simulink model "BANSHEE"  (Simulink 8.1)
settings: Solver=ode1  StartTime=0.0  StopTime=inf  FixedStep=Ts  MaxStep=1e-3  RelTol=1e-3
model workspace (MAT data in the model file):
  op_snapshot1 : opcond.OperatingPoint (value not decoded)
PostLoadFcn:
  | BANSHEE_init;
InitFcn:
  | BANSHEE_init;
values from neighbouring files (symbols this model uses):
  Ts = 100E-6    (= 0.0001)    [BANSHEE_init.m]
undefined symbols (not defined in the file or in its folder): Banshee_HWCtrl_IOs, Banshee_SEL751_Woodward_lib, DMS_slave_lib, DMSCommands, F1, F2, F3, fdesignblkfcn, Feeder1_lib, Feeder2_lib, Feeder3_lib, gcbh, generic_ethernet_cb, Left, relay_housing_lib, SM_UtilityService, SS_F1_RELAY_HOUSING, SS_F2_RELAY_HOUSING, SS_F3_RELAY_HOUSING, SS_Feeder1, SS_Feeder2, SS_Feeder3, TestSeq_slave_lib, TestSequenceCommands, type, utility_service_lib, V
libraries: breaker_lib x51, cables_lib x49, rtio_generic_modbus x45, relay_modbus_lib x42, transformer_lib x25, rtlab x23, simulink x23, Load_lib x20, powerlib x19, ssn_lib x17, rtio_opalrt_common x13, rtio_opalrt_op5142ex1 x12
(part 1 of 6)
settings Model: ARTEMISmethode_block_infos=$$__separator__$$BANSHEE/ARTEMIS Guide$$__separator__$$  Creator=RE25624  LastModifiedBy=re25624  BufferReuse=off
settings SolverCC: ZeroCrossAlgorithm=Adaptive
settings DataIOCC: ExternalInput=getinputstruct(op_snapshot1)  InitialState=getstatestruct(op_snapshot1)  LimitDataPoints=off  MaxDataPoints=90060  SignalLoggingSaveFormat=Dataset  SaveOutput=off  SignalLogging=off  DSMLogging=off  SaveTime=off  OutputSaveName=result
settings OptimizationCC: BlockReduction=off  OptimizeBlockIOStorage=off  BufferReuse=off  ExpressionFolding=off  LocalBlockOutputs=off
settings DebuggingCC: MaxConsecutiveZCsMsg=warning  IgnoredZcDiagnostic=none  SolverPrmCheckMsg=none  MultiTaskRateTransMsg=warning  FcnCallInpInsideContextMsg=EnableAllAsWarning  FrameProcessingCompatibilityMsg=error  ModelReferenceExtraNoncontSigs=warning  StrictBusMsg=None
settings ModelReferenceCC: UpdateModelReferenceTargets=IfOutOfDate
settings SFSimCC: SFSimEcho=off
settings GRTTargetCC: CodeReplacementLibrary=C89/C90 (ANSI)

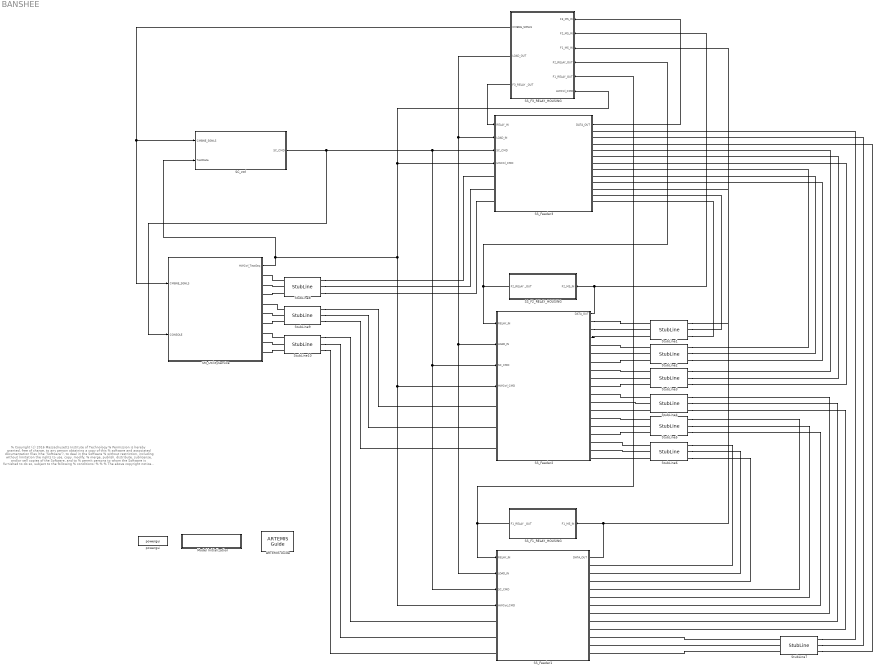
== system BANSHEE ==
  note: % Copyright (c) 2016 Massachusetts Institute of Technology
      | % Permission is hereby granted, free of charge, to any person obtaining a copy of this
      | % software and associated documentation files (the "Software"), to deal in the Software
      | % without restriction, including without limitation the rights to use, copy, modify,
      | % merge, publish, distribute, sublicense, and/or sell copies of the Software, and to
      | % permit persons to whom the Software is furnished to do so, subject to the following
      | % conditions:
      | %
      | %
      | % The above copyright notice and this permission notice shall be included in
      | % all copies or substantial portions of the Software.
      | %
      | % THE SOFTWARE IS PROVIDED "AS IS", WITHOUT WARRANTY OF ANY KIND, EXPRESS OR IMPLIED,
      | % INCLUDING BUT NOT LIMITED TO THE WARRANTIES OF MERCHANTABILITY, FITNESS FOR A
      | % PARTICULAR PURPOSE AND NONINFRINGEMENT. IN NO EVENT SHALL THE AUTHORS OR COPYRIGHT
      | % HOLDERS BE LIABLE FOR ANY CLAIM, DAMAGES OR OTHER LIABILITY, WHETHER IN AN ACTION
      | % OF CONTRACT, TORT OR OTHERWISE, ARISING FROM, OUT OF OR IN CONNECTION WITH THE
      | % SOFTWARE OR THE USE OR OTHER DEALINGS IN THE SOFTWARE.
      | %
      | %
      | %%
  ARTEMIS Guide : artemis/ARTEMIS/ARTEMIS Guide  Tag=FTSSmethode_opal_4hx0r99  Description=5.0_z1  lock=on  Ts=Ts  opt=art5  dyna=off  nb_perm=4  RT_fullcomp=off  ssn=on  ssn_itvc=off  ssn_ivic=off  ssn_ext=off  ssn_solver=Art5 with Backward Euler nodal interface  ssn_impulse=off  ssn_quasimpulse=off  ssn_impulse_loop=5  paraExtinctionThy=off  Thy_Impulse=on  dtc=Off  dtc_opt=normal  ao=on  simtype=off  ct_mac=off  lin_mov=off  lsp=[0.001 2]  spike_skip=Disabled  dtc_extra=1  dtc_sws=normal  dtc_pied=0.5  SPSRulesBlock=SPSRules  tre=on  ctmm=off  LF=off  dpl_type=ARTEMiS DPL  rlc_type=off  custom_type=off  para=on  ssn_ImpulseLoopBlockedStateUpdate=5  ssn_mov_iter_number=5  ssn_switch_iter_number=5
  Model Initialization : Subsystem  AncestorBlock=artemis/Tools /Misc/Model Initialization  mask(Model Functions){InitFcnX=BANSHEE_init;, prel=off, posl=on, inif=on, strf=off}
      mask prompts: InitFcnX "Initialisation"; prel "Preload Function"; posl "PostLoad Function"; inif "InitFcn"; strf "StartFcn"
      mask init:
      | currentBlock = gcb;
      | root = bdroot(currentBlock);
      | 
      | if ~strcmp(get_param(root,'BlockDiagramType'),'library')
      |     if prel==1
      |         set_param(root, 'PreLoadFcn', InitFcnX);
      |     else
      |         set_param(root, 'PreLoadFcn', '');
      |     end
      |     if inif==1
      |         set_param(root, 'InitFcn', InitFcnX);
      |     else
      |         set_param(root, 'InitFcn', '');
      |     end
      |     if strf==1
      |         set_param(root, 'StartFcn', InitFcnX);
      |     else
      |         set_param(root, 'StartFcn', '');
      |     end
      |     if posl==1
      |         set_param(root, 'PostLoadFcn', InitFcnX);
      |     else
      |         set_param(root, 'PostLoadFcn', '');
      |     end
      | end
      | 
      | pos = get_param(currentBlock, 'Position');
      | width = pos(3) - pos(1); height = pos(4) - pos(2);
      | txt = [ upper(root) '\n' '- InitFcn. . . . . '  get_param(root, 'InitFcn') ];
      settings: CopyFcn=set_param(gcb,'LinkStatus','inactive')
      mask Display: text(5, height*0.5, txt, 'horizontalAlignment', 'left', 'verticalAlignment', 'middle') ;
  SC_ctrl : Subsystem
  SM_UtilityService : Subsystem  AncestorBlock=utility_service_lib/SM_UtilityService
  SS_F1_RELAY_HOUSING : Subsystem  AncestorBlock=relay_housing_lib/SS_F1_RELAY_HOUSING
  SS_F2_RELAY_HOUSING : Subsystem  AncestorBlock=relay_housing_lib/SS_F2_RELAY_HOUSING
  SS_F3_RELAY_HOUSING : Subsystem  AncestorBlock=relay_housing_lib/SS_F3_RELAY_HOUSING
  SS_Feeder1 : Subsystem  AncestorBlock=Feeder1_lib/SS_Feeder1
  SS_Feeder2 : Subsystem  AncestorBlock=Feeder2_lib/SS_Feeder2
  SS_Feeder3 : Subsystem  AncestorBlock=Feeder3_lib/SS_Feeder3
  StubLine1 : artemis/ARTEMIS/StubLine  Phases=3  pu=off  L=1500 * 9.43453e-08 / 2  Lpu=0.08  R=1500 * 2.28409e-5 / 2  Rpu=0.002  S_base=450e6/3  V_base=230e3/sqrt(3)  F_base=60  Ts=Ts
  StubLine10 : artemis/ARTEMIS/StubLine  Phases=3  pu=on  L=1500 * 9.43453e-08 / 2  Lpu=0.08  R=1500 * 2.28409e-5 / 2  Rpu=0.002  S_base=50e6/3  V_base=13.8e3/sqrt(3)  F_base=60  Ts=Ts
  StubLine2 : artemis/ARTEMIS/StubLine  Phases=3  pu=off  L=1500 * 9.43453e-08 / 2  Lpu=0.08  R=1500 * 2.28409e-5 / 2  Rpu=0.002  S_base=450e6/3  V_base=230e3/sqrt(3)  F_base=60  Ts=Ts
  StubLine3 : artemis/ARTEMIS/StubLine  Phases=3  pu=off  L=1500 * 9.43453e-08 / 2  Lpu=0.08  R=1500 * 2.28409e-5 / 2  Rpu=0.002  S_base=450e6/3  V_base=230e3/sqrt(3)  F_base=60  Ts=Ts
  StubLine4 : artemis/ARTEMIS/StubLine  Phases=3  pu=off  L=1000 * 9.43453e-08 / 2  Lpu=0.08  R=1000 * 2.28409e-5 / 2  Rpu=0.002  S_base=450e6/3  V_base=230e3/sqrt(3)  F_base=60  Ts=Ts
  StubLine5 : artemis/ARTEMIS/StubLine  Phases=3  pu=off  L=2000 * 9.43453e-08 / 2  Lpu=0.08  R=2000 * 2.28409e-5 / 2  Rpu=0.002  S_base=450e6/3  V_base=230e3/sqrt(3)  F_base=60  Ts=Ts
  StubLine6 : artemis/ARTEMIS/StubLine  Phases=3  pu=off  L=3000 * 9.43453e-08 / 1  Lpu=0.08  R=3000 * 2.28409e-5 / 1  Rpu=0.002  S_base=450e6/3  V_base=230e3/sqrt(3)  F_base=60  Ts=Ts
  StubLine7 : artemis/ARTEMIS/StubLine  Phases=3  pu=off  L=2000 * 9.43453e-08 / 2  Lpu=0.08  R=2000 * 2.28409e-5 / 2  Rpu=0.002  S_base=450e6/3  V_base=230e3/sqrt(3)  F_base=60  Ts=Ts
  StubLine8 : artemis/ARTEMIS/StubLine  Phases=3  pu=on  L=1500 * 9.43453e-08 / 2  Lpu=0.08  R=1500 * 2.28409e-5 / 2  Rpu=0.002  S_base=50e6/3  V_base=13.8e3/sqrt(3)  F_base=60  Ts=Ts
  StubLine9 : artemis/ARTEMIS/StubLine  Phases=3  pu=on  L=1500 * 9.43453e-08 / 2  Lpu=0.08  R=1500 * 2.28409e-5 / 2  Rpu=0.002  S_base=50e6/3  V_base=13.8e3/sqrt(3)  F_base=60  Ts=Ts
  powergui : powerlib/powergui  Priority=2  SimulationMode=Discrete  SolverType=Tustin  SampleTime=Ts  frequency=60  SPID=off  DisableSnubberDevices=off  DisableRonSwitches=off  DisableVfSwitches=off  SwTol=0  Interpol=off  DisplayEquations=off  frequencyindice=0  Pbase=100e6  ErrMax=1e-4  Iterations=50  UnitsV=kV  UnitsW=MW  FunctionMessages=off  echomessages=off  HookPort=off  EnableUseOfTLC=off  x0status=blocks  RestoreLinks=warning  ResistiveCurrentMeasurement=off  Frange=logspace(0,3,50)  Ylog=off  Xlog=off  ShowGrid=off  save=off  variable=ZData  structure=0  ZoomFFT=on  StartTime=0.0  cycles=2  DisplayStyle=off  fundamental=60  FreqAxis=off  MaxFrequency=1000  frequencyindicesteady=1  RmsSteady=1  display=off  Ts=0  methode=off
  wires:
  SS_Feeder3/1(DATA_OUT) -> SS_F3_RELAY_HOUSING/1(F3_MS_IN)
  SS_F3_RELAY_HOUSING/3(F3_RELAY _OUT) -> SS_Feeder3/1(RELAY_IN)
  SS_F1_RELAY_HOUSING/1(F1_RELAY _OUT) -> SS_Feeder1/1(RELAY_IN), SS_F3_RELAY_HOUSING/5(F1_RELAY_OUT)
  SS_F2_RELAY_HOUSING/1(F2_RELAY _OUT) -> SS_F3_RELAY_HOUSING/4(F2_RELAY_OUT), SS_Feeder2/1(RELAY_IN)
  SS_Feeder1/1(DATA_OUT) -> SS_F3_RELAY_HOUSING/3(F1_MS_IN), SS_F1_RELAY_HOUSING/1(F1_MS_IN)
  SS_Feeder2/1(DATA_OUT) -> SS_F3_RELAY_HOUSING/2(F2_MS_IN), SS_F2_RELAY_HOUSING/1(F2_MS_IN)
  SS_F3_RELAY_HOUSING/2(LOAD_OUT) -> SS_Feeder1/2(LOAD_IN), SS_Feeder2/2(LOAD_IN), SS_Feeder3/2(LOAD_IN)
  SM_UtilityService/1(HWCtrl_TestSeq) -> SC_ctrl/2(TestData), SS_Feeder1/4(HWCtrl_CMD), SS_Feeder2/4(HWCtrl_CMD), SS_F3_RELAY_HOUSING/6(HWCtrl_CMD), SS_Feeder3/4(HWCtrl_CMD)
  SS_F3_RELAY_HOUSING/1(CMBNE_SGNLS) -> SM_UtilityService/1(CMBNE_SGNLS), SC_ctrl/1(CMBNE_SGNLS)
  SC_ctrl/1(SC_CMD) -> SS_Feeder1/3(SC_CMD), SS_Feeder2/3(SC_CMD), SS_Feeder3/3(SC_CMD), SM_UtilityService/2(CONSOLE)
  connections:
  SS_Feeder2/RConn2 -- StubLine1/LConn2
  SS_Feeder2/RConn1 -- StubLine1/LConn1
  SS_Feeder2/RConn3 -- StubLine1/LConn3
  StubLine2/LConn2 -- SS_Feeder2/RConn5
  StubLine2/LConn3 -- SS_Feeder2/RConn6
  StubLine2/LConn1 -- SS_Feeder2/RConn4
  StubLine3/LConn2 -- SS_Feeder2/RConn8
  StubLine3/LConn1 -- SS_Feeder2/RConn7
  StubLine3/LConn3 -- SS_Feeder2/RConn9
  StubLine4/LConn3 -- SS_Feeder2/RConn12
  StubLine4/LConn2 -- SS_Feeder2/RConn11
  StubLine4/LConn1 -- SS_Feeder2/RConn10
  StubLine7/LConn3 -- SS_Feeder1/RConn12
  StubLine7/LConn2 -- SS_Feeder1/RConn11
  StubLine7/LConn1 -- SS_Feeder1/RConn10
  StubLine5/LConn2 -- SS_Feeder2/RConn14
  StubLine5/LConn1 -- SS_Feeder2/RConn13
  StubLine5/LConn3 -- SS_Feeder2/RConn15
  StubLine6/LConn3 -- SS_Feeder2/RConn18
  StubLine6/LConn2 -- SS_Feeder2/RConn17
  StubLine6/LConn1 -- SS_Feeder2/RConn16
  StubLine6/RConn1 -- SS_Feeder1/RConn1
  StubLine6/RConn2 -- SS_Feeder1/RConn2
  StubLine6/RConn3 -- SS_Feeder1/RConn3
  StubLine5/RConn1 -- SS_Feeder1/RConn4
  StubLine5/RConn2 -- SS_Feeder1/RConn5
  StubLine5/RConn3 -- SS_Feeder1/RConn6
  StubLine4/RConn1 -- SS_Feeder1/RConn7
  StubLine4/RConn2 -- SS_Feeder1/RConn8
  StubLine4/RConn3 -- SS_Feeder1/RConn9
  StubLine3/RConn3 -- SS_Feeder3/RConn6
  StubLine3/RConn2 -- SS_Feeder3/RConn5
  StubLine3/RConn1 -- SS_Feeder3/RConn4
  StubLine2/RConn3 -- SS_Feeder3/RConn9
  StubLine2/RConn2 -- SS_Feeder3/RConn8
  StubLine2/RConn1 -- SS_Feeder3/RConn7
  StubLine1/RConn3 -- SS_Feeder3/RConn12
  StubLine1/RConn2 -- SS_Feeder3/RConn11
  StubLine1/RConn1 -- SS_Feeder3/RConn10
  StubLine7/RConn1 -- SS_Feeder3/RConn1
  StubLine7/RConn2 -- SS_Feeder3/RConn2
  StubLine7/RConn3 -- SS_Feeder3/RConn3
  StubLine8/LConn1 -- SM_UtilityService/RConn1
  StubLine8/LConn2 -- SM_UtilityService/RConn2
  StubLine8/LConn3 -- SM_UtilityService/RConn3
  StubLine9/LConn2 -- SM_UtilityService/RConn5
  StubLine9/LConn3 -- SM_UtilityService/RConn6
  StubLine9/LConn1 -- SM_UtilityService/RConn4
  StubLine10/LConn2 -- SM_UtilityService/RConn8
  StubLine10/LConn3 -- SM_UtilityService/RConn9
  StubLine10/LConn1 -- SM_UtilityService/RConn7
  StubLine8/RConn3 -- SS_Feeder3/LConn3
  StubLine8/RConn2 -- SS_Feeder3/LConn2
  StubLine8/RConn1 -- SS_Feeder3/LConn1
  StubLine10/RConn1 -- SS_Feeder1/LConn1
  StubLine10/RConn2 -- SS_Feeder1/LConn2
  StubLine10/RConn3 -- SS_Feeder1/LConn3
  StubLine9/RConn1 -- SS_Feeder2/LConn1
  StubLine9/RConn2 -- SS_Feeder2/LConn2
  StubLine9/RConn3 -- SS_Feeder2/LConn3

== system BANSHEE/Model Initialization ==

== system BANSHEE/SC_ctrl ==
  note: % Copyright (c) 2016 Massachusetts Institute of Technology
      | % Permission is hereby granted, free of charge, to any person obtaining a copy of this
      | % software and associated documentation files (the "Software"), to deal in the Software
      | % without restriction, including without limitation the rights to use, copy, modify,
      | % merge, publish, distribute, sublicense, and/or sell copies of the Software, and to
      | % permit persons to whom the Software is furnished to do so, subject to the following
      | % conditions:
      | %
      | %
      | % The above copyright notice and this permission notice shall be included in
      | % all copies or substantial portions of the Software.
      | %
      | % THE SOFTWARE IS PROVIDED "AS IS", WITHOUT WARRANTY OF ANY KIND, EXPRESS OR IMPLIED,
      | % INCLUDING BUT NOT LIMITED TO THE WARRANTIES OF MERCHANTABILITY, FITNESS FOR A
      | % PARTICULAR PURPOSE AND NONINFRINGEMENT. IN NO EVENT SHALL THE AUTHORS OR COPYRIGHT
      | % HOLDERS BE LIABLE FOR ANY CLAIM, DAMAGES OR OTHER LIABILITY, WHETHER IN AN ACTION
      | % OF CONTRACT, TORT OR OTHERWISE, ARISING FROM, OUT OF OR IN CONNECTION WITH THE
      | % SOFTWARE OR THE USE OR OTHER DEALINGS IN THE SOFTWARE.
      | %
      | %
      | %%
  CMBNE_SGNLS : Inport
  TestData : Inport  Port=2
  Bus Creator : BusCreator  Inputs=2
  Bus Creator1 : BusCreator  Inputs=5
  Bus Creator2 : BusCreator  Inputs=2
  Bus Creator3 : BusCreator  Inputs=5
  DO NOT WRITE : Constant  Value=0
  F1 1: connect motor 0: disconnect motor1 : Constant  Value=0
  F3 1: connect motor 0: disconnect motor : Constant  Value=0
  FAULT : Constant
  Grid_Status_Ctrl : Subsystem  mask(Grid Status Control){Substation=1, Grid_F1=1, Grid_F2=1, Grid_F3=1, useDTT=1}
      mask prompts: Substation "Substation On [1] - Off [0]"; Grid_F1 "Grid_F1 On [1] - Off [0]"; Grid_F2 "Grid_F2 On [1] - Off [0]"; Grid_F3 "Grid_F3 On [1] - Off [0]"; useDTT "DTT Active On [1] - Off [0]"
      mask help: Use this block to trip and reconnect the feeder breakers serving Banshee
  Manual Switch{,1..6} (7 alike) : ManualSwitch
  NO FAULT : Constant  Value=0
  OpComm : rtlab/OpComm  nbport=2  groupe_acq=1  subsys_rate=0  st=0  Synchronization=on  Interpolation=on  Threshold=1.0  Missed_Data=off  Sim_Time=off  Samples=off  dynSigOut=off  from_console=0  warning_done=off  writeOpCommFile=off  Offset=off
  Plots : Subsystem
  Status : Display
  TestSeq : Subsystem
  WRITE : Constant
  Woodward : Subsystem
  SC_CMD : Outport
  wires:
  CMBNE_SGNLS/1 -> OpComm/1
  Bus Creator1/1 -> SC_CMD/1
  [IO_ctrl] -> Bus Creator1/3  "IO ctrl"
  Woodward/1(IOctrl) -> [IO_ctrl]
  [fault_cmd] -> Bus Creator1/1  "fault_cmd"
  Bus Creator/1 -> Bus Creator1/2  "motor_ONOFF"
  F3 1: connect motor 0: disconnect motor/1 -> Bus Creator/1  "F3_motor_ONOFF"
  F1 1: connect motor 0: disconnect motor1/1 -> Bus Creator/2  "F1_motor_ONOFF"
  Grid_Status_Ctrl/1(o) -> Status/1, Bus Creator1/4  "GridStatusCtrl"
  Manual Switch/1 -> Bus Creator2/1  "record_rms_signals"
  Manual Switch1/1 -> Bus Creator2/2  "record_inst_signals"
  Bus Creator2/1 -> Bus Creator1/5  "DataLogging"
  OpComm/1 -> Plots/1(CMBNE_SGNLS)
  OpComm/2 -> TestSeq/1(TestData)
  TestData/1 -> OpComm/2
  WRITE/1 -> Manual Switch1/2, Manual Switch/2  "record_rms_signals"
  DO NOT WRITE/1 -> Manual Switch1/1, Manual Switch/1
  Bus Creator3/1 -> [fault_cmd]
  Manual Switch2/1 -> Bus Creator3/1  "fault_location_1"
  Manual Switch6/1 -> Bus Creator3/5  "fault_location_5"
  Manual Switch3/1 -> Bus Creator3/2  "fault_location_2"
  Manual Switch4/1 -> Bus Creator3/3  "fault_location_3"
  Manual Switch5/1 -> Bus Creator3/4  "fault_location_4"
  NO FAULT/1 -> Manual Switch6/1, Manual Switch5/1, Manual Switch4/1, Manual Switch3/1, Manual Switch2/1
  FAULT/1 -> Manual Switch2/2, Manual Switch6/2, Manual Switch5/2, Manual Switch4/2, Manual Switch3/2  "record_rms_signals"

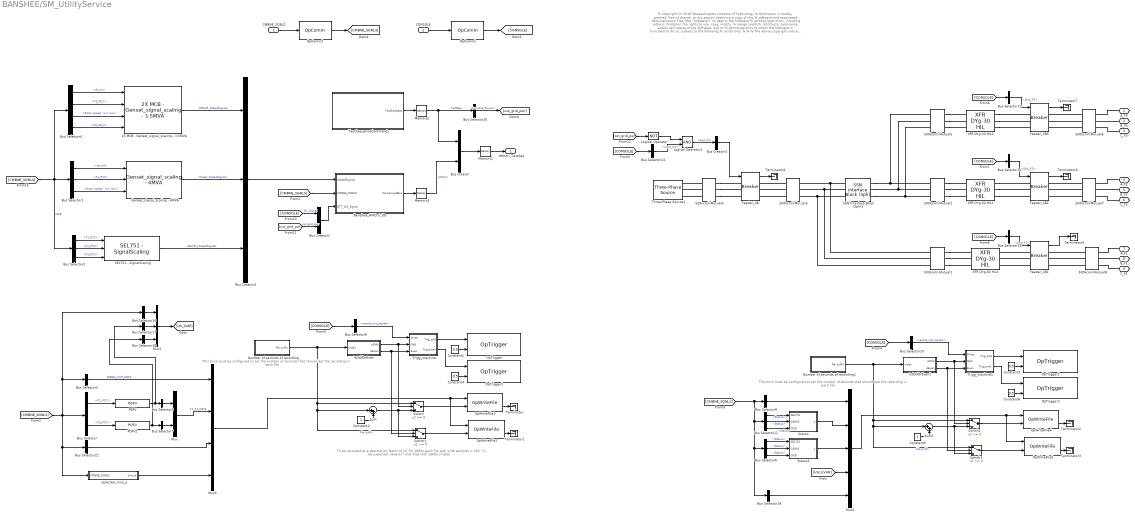
== system BANSHEE/SM_UtilityService ==
  note: % Copyright (c) 2016 Massachusetts Institute of Technology
      | % Permission is hereby granted, free of charge, to any person obtaining a copy of this
      | % software and associated documentation files (the "Software"), to deal in the Software
      | % without restriction, including without limitation the rights to use, copy, modify,
      | % merge, publish, distribute, sublicense, and/or sell copies of the Software, and to
      | % permit persons to whom the Software is furnished to do so, subject to the following
      | % conditions:
      | %
      | %
      | % The above copyright notice and this permission notice shall be included in
      | % all copies or substantial portions of the Software.
      | %
      | % THE SOFTWARE IS PROVIDED "AS IS", WITHOUT WARRANTY OF ANY KIND, EXPRESS OR IMPLIED,
      | % INCLUDING BUT NOT LIMITED TO THE WARRANTIES OF MERCHANTABILITY, FITNESS FOR A
      | % PARTICULAR PURPOSE AND NONINFRINGEMENT. IN NO EVENT SHALL THE AUTHORS OR COPYRIGHT
      | % HOLDERS BE LIABLE FOR ANY CLAIM, DAMAGES OR OTHER LIABILITY, WHETHER IN AN ACTION
      | % OF CONTRACT, TORT OR OTHERWISE, ARISING FROM, OUT OF OR IN CONNECTION WITH THE
      | % SOFTWARE OR THE USE OR OTHER DEALINGS IN THE SOFTWARE.
      | %
      | %
      | %%
  note: This bock must be configured to set the number of
      | seconds that should last the recording in each file
  note: To be recorded at a decimation factor of 10,   for 1800s each file with a Nb samples = 200.
      | To be expected: several *.mat files with 1800s of data
  note: This bock must be configured to set the number of
      | seconds that should last the recording in each file
  CMBNE_SGNLS : Inport
  CONSOLE : Inport  Port=2
  2X MCB - Genset_signal_scaling - 3.5MVA : EasyGen3500_GensetSignalScaling_lib/2X MCB - Genset_signal_scaling - 3.5MVA  Vpk_mcb=11268  watt_mcb=3150000  Vpk_gcb=11268  watt_gcb=3150000  rated_rpm=1800  wm_noise_bias=0.02
  500kcmil-Mutual1 : cables_lib/500kcmil-Mutual  length=200  par_sets=1  ratio=3
  500kcmil-Mutual2 : cables_lib/500kcmil-Mutual  length=200  par_sets=1  ratio=3
  500kcmil-Mutual{3..4,6..8} (5 alike) : cables_lib/500kcmil-Mutual  length=50  par_sets=1  ratio=3
  500kcmil-Mutual5 : cables_lib/500kcmil-Mutual  length=200  par_sets=1  ratio=3
  Banshee_HWCtrl_IOs : Subsystem  AncestorBlock=Banshee_SEL751_Woodward_lib/Banshee_HWCtrl_IOs
  Bus Creator : BusCreator  Inputs=2
  Bus Creator1 : BusCreator  Inputs=2
  Bus Creator2 : BusCreator  Inputs=1
  Bus Creator4 : BusCreator  Inputs=3
  Bus Selector : BusSelector  OutputSignals=F1_MS_IN.CB_DATA.F1_PCC,F3_MS_IN.CB_DATA.F3_PCC
  Bus Selector1 : BusSelector  OutputSignals="F1_MS_IN.DIESEL_DATA.DIESEL_GCB.cb_ms,F1_MS_IN.CB_DATA.F1_PCC,F1_MS_IN.DIESEL_DATA.Gen2_meas.w.w.Rotor speed  wm (pu)"
  Bus Selector10 : BusSelector  OutputSignals=DataLogging.record_inst_signals
  Bus Selector11 : BusSelector  OutputSignals=F1_MS_IN.CB_DATA.F1_PCC.Status,F1_MS_IN.CB_DATA.F1_CB_3.Status,F1_MS_IN.DIESEL_DATA.DIESEL_GCB.cb_ms.Status
  Bus Selector12 : BusSelector  OutputSignals=GridStatusCtrl.Substation.Logic_trip
  Bus Selector13 : BusSelector  OutputSignals=GridStatusCtrl.Grid_F3
  Bus Selector14 : BusSelector  OutputSignals=GridStatusCtrl.Grid_F2
  Bus Selector15 : BusSelector  OutputSignals=GridStatusCtrl.Grid_F1
  Bus Selector16 : BusSelector  OutputSignals=F1_MS_IN.DIESEL_DATA.DIESEL_GCB.kw,F1_MS_IN.DIESEL_DATA.DIESEL_GCB.kvar,F3_MS_IN.NG_CHP_DATA.NG_CHP_GCB.kw,F3_MS_IN.NG_CHP_DATA.NG_CHP_GCB.kvar  OutputAsBus=on
  Bus Selector17 : BusSelector  OutputSignals=kw,kvar  OutputAsBus=on
  Bus Selector18 : BusSelector  OutputSignals=kw,kvar  OutputAsBus=on
  Bus Selector19 : BusSelector  OutputSignals=F1_MS_IN.DIESEL_DATA.DIESEL_GCB.cb_ms.Iabc,F3_MS_IN.NG_CHP_DATA.NG_CHP_GCB.cb_ms.Iabc,F1_MS_IN.DIESEL_DATA.Gen2_meas.Vf.vf,F3_MS_IN.NG_CHP_DATA.Gen1_meas.Vf.vf  OutputAsBus=on
  Bus Selector2 : BusSelector  OutputSignals=F1_MS_IN.CB_DATA.F1_PCC,F2_MS_IN.CB_DATA.F2_PCC,F3_MS_IN.CB_DATA.F3_PCC
  Bus Selector20 : BusSelector  OutputSignals=Cut_Grid_Power
  Bus Selector21 : BusSelector  OutputSignals=F1_RELAY_OUT.F1_CB_1.m.status,F1_RELAY_OUT.F1_CB_2.m.status,F1_RELAY_OUT.F1_CB_3.m.status,F1_RELAY_OUT.F1_CB_4.m.status,F1_RELAY_OUT.F1_CB_5.m.status,F1_RELAY_OUT.F1_CB_6.m.status,F1_RELAY_OUT.F1_CB_7.m.status,F1_RELAY_OUT.F1_CB_8.m.status,F1_RELAY_OUT.F1_CB_9.m.status,F1_RELAY_OUT.F1_CB_10.m.status,F1_RELAY_OUT.F1_CB_11.m.status,F1_RELAY_OUT.F1_CB_12.m.status,F1_RELAY_OUT.F1_CB_13.m.status,F1_RELAY_OUT.F1_CB_14.m.status,F2_RELAY_OUT.F2_CB_1.m.status,F2_RELAY_OUT.F2_CB_2.m.status,F2_RELAY_OUT.F2_CB_3.m.status,F2_RELAY_OUT.F2_CB_4.m.status,F2_RELAY_OUT.F2_CB_5.m.status,F2_RELAY_OUT.F2_CB_6.m.status,F2_RELAY_OUT.F2_CB_7.m.status,F2_RELAY_OUT.F2_CB_8.m.status,F2_RELAY_OUT.F2_CB_9.m.status,F2_RELAY_OUT.F2_CB_10.m.status,F2_RELAY_OUT.F2_CB_11.m.status,F2_RELAY_OUT.F2_CB_12.m.status,F2_RELAY_OUT.F2_CB_13.m.status,F2_RELAY_OUT.F2_CB_14.m.status,F2_RELAY_OUT.F2_CB_15.m.status,F2_RELAY_OUT.F2_CB_16.m.status,F2_RELAY_OUT.F2_CB_17.m.status,F2_RELAY_OUT.F2_CB_18.m.status,F2_RELAY_OUT.F2_CB_19.m.status,F3_RELAY_OUT.F3_CB_1.m.status,F3_RELAY_OUT.F3_CB_2.m.status,F3_RELAY_OUT.F3_CB_3.m.status,F3_RELAY_OUT.F3_CB_4.m.status,F3_RELAY_OUT.F3_CB_5.m.status,F3_RELAY_OUT.F3_CB_6.m.status,F3_RELAY_OUT.F3_CB_7.m.status,F3_RELAY_OUT.F3_CB_8.m.status,F3_RELAY_OUT.F3_CB_9.m.status  OutputAsBus=on
  Bus Selector3 : BusSelector  OutputSignals=F1_MS_IN.DIESEL_DATA.DIESEL_GCB.VRMSLL,F1_MS_IN.DIESEL_DATA.DIESEL_GCB.Freq,F1_MS_IN.DIESEL_DATA.DIESEL_GCB.kw,F1_MS_IN.DIESEL_DATA.DIESEL_GCB.kvar,F3_MS_IN.NG_CHP_DATA.NG_CHP_GCB.VRMSLL,F3_MS_IN.NG_CHP_DATA.NG_CHP_GCB.Freq,F3_MS_IN.NG_CHP_DATA.NG_CHP_GCB.kw,F3_MS_IN.NG_CHP_DATA.NG_CHP_GCB.kvar  OutputAsBus=on
  Bus Selector4 : BusSelector  OutputSignals="F3_MS_IN.NG_CHP_DATA.NG_CHP_GCB.cb_ms,F3_MS_IN.CB_DATA.F3_PCC,F3_MS_IN.NG_CHP_DATA.Gen1_meas.w.w.Rotor speed  wm (pu),F3_MS_IN.CB_DATA.F3_CB_3"
  Bus Selector5 : BusSelector  OutputSignals=VRMSLL,Freq,kw,kvar  OutputAsBus=on
  Bus Selector6 : BusSelector  OutputSignals=F3_MS_IN.CB_DATA.F3_PCC.Status,F3_MS_IN.CB_DATA.F3_CB_3.Status,F3_MS_IN.NG_CHP_DATA.NG_CHP_GCB.cb_ms.Status
  Bus Selector7 : BusSelector  OutputSignals=VRMSLL,Freq,kw,kvar  OutputAsBus=on
  Bus Selector8 : BusSelector  OutputSignals=DataLogging.record_rms_signals
  Bus Selector9 : BusSelector  OutputSignals=F1_MS_IN.CB_DATA.F1_PCC.Vabc_bus,F3_MS_IN.CB_DATA.F3_PCC.Vabc_bus,F1_MS_IN.DIESEL_DATA.DIESEL_GCB.cb_ms.Vabc_bus,F3_MS_IN.NG_CHP_DATA.NG_CHP_GCB.cb_ms.Vabc_bus  OutputAsBus=on
  Constant{1,3..4,6} (4 alike) : Constant  Value=0.5
  Constant2 : Constant
  Constant5 : Constant
  Feeder_CB{,1..3} (4 alike) : breaker_lib/Breaker  Ts=Ts  mech_delay=cb_mech_delay
  Genset_signal_scaling - 4MVA : EasyGen3500_GensetSignalScaling_lib/Genset_signal_scaling - 4MVA  Vpk_mcb=11268  watt_mcb=3600000  Vpk_gcb=11268  watt_gcb=3600000  rated_rpm=1800  wm_noise_bias=0.02
  Logical Operator : Logic  Operator=NOT  AllPortsSameDT=off  OutDataTypeStr=boolean
  Logical Operator1 : Logic  AllPortsSameDT=off  OutDataTypeStr=boolean
  Memory1 : Memory
  Memory2 : Memory
  Memory3 : Memory
  Mux : Mux  Inputs=2
  Mux1 : Mux  Inputs=3
  Mux2 : Mux  Inputs=5
  Mux3 : Mux
  Number of seconds of recording : Subsystem  mask{time_s=1800}
      mask prompts: time_s "Time in seconds"
      mask help: Set the number of seconds that should last the recording in each file.
  Number of seconds of recording1 : Subsystem  mask{time_s=300}
      mask prompts: time_s "Time in seconds"
      mask help: Set the number of seconds that should last the recording in each file.
  OpComm1 : rtlab/OpComm  nbport=1  groupe_acq=1  subsys_rate=0  st=0  Synchronization=on  Interpolation=on  Threshold=1.0  Missed_Data=off  Sim_Time=off  Samples=off  dynSigOut=off  from_console=1  warning_done=off  writeOpCommFile=off  Offset=off
  OpComm2 : rtlab/OpComm  nbport=1  groupe_acq=1  subsys_rate=0  st=0  Synchronization=on  Interpolation=on  Threshold=1.0  Missed_Data=off  Sim_Time=off  Samples=off  dynSigOut=off  from_console=0  warning_done=off  writeOpCommFile=off  Offset=off
  OpTrigger : rtlab/DataLogging/OpTrigger  Trig_Type=TRIGGER SIGNAL >= TRIGGER LEVEL  Trig_Offset=0  Acq_Group=28
  OpTrigger1 : rtlab/DataLogging/OpTrigger  Trig_Type=TRIGGER SIGNAL >= TRIGGER LEVEL  Trig_Offset=0  Acq_Group=29
  OpTrigger2 : rtlab/DataLogging/OpTrigger  Trig_Type=TRIGGER SIGNAL >= TRIGGER LEVEL  Trig_Offset=0  Acq_Group=26
  OpTrigger3 : rtlab/DataLogging/OpTrigger  Trig_Type=TRIGGER SIGNAL >= TRIGGER LEVEL  Trig_Offset=0  Acq_Group=27
  OpWriteFile1 : rtlab/DataLogging/OpWriteFile  Static_File=off  varname=recVar  Filename=A_FILE_RECORDED_o.mat  rtpath='./'  nrtpath='.\'  Acq_Group=28  file_size=150000000  write_offline=off  Sim_Mode=off  Nb_Samples=1000  Buffer_size=0
      settings: Decimation=20
  OpWriteFile2 : rtlab/DataLogging/OpWriteFile  Static_File=off  varname=recVar  Filename=A_FILE_RECORDED_e.mat  rtpath='./'  nrtpath='.\'  Acq_Group=29  file_size=150000000  write_offline=off  Sim_Mode=off  Nb_Samples=1000  Buffer_size=0
      settings: Decimation=20
  OpWriteFile4 : rtlab/DataLogging/OpWriteFile  Static_File=off  varname=recVar  Filename=A_INST_RECORDED_o.mat  rtpath='./'  nrtpath='.\'  Acq_Group=26  file_size=150000000  write_offline=off  Sim_Mode=off  Nb_Samples=1000  Buffer_size=0
      settings: Decimation=4
  OpWriteFile5 : rtlab/DataLogging/OpWriteFile  Static_File=off  varname=recVar  Filename=A_INST_RECORDED_e.mat  rtpath='./'  nrtpath='.\'  Acq_Group=27  file_size=150000000  write_offline=off  Sim_Mode=off  Nb_Samples=1000  Buffer_size=0
      settings: Decimation=4
  PQFV : PQFV_lib/PQFV  VRMSLL=13800
  PQFV2 : PQFV_lib/PQFV  VRMSLL=13800
  SEL751 - SignalScaling : SEL751_SignalScaling_lib/SEL751 - SignalScaling  ct_ratio=1/1250  pt_ratio=1/1800
  SSN Interface Block (3ph)3 : ssn_lib/SSN Interface Block (3ph)  nb_phase=3  nb_port=2  p1_type=V-type(Left)  p2_type=V-type (Right)  p3_type=V-type(Left)  p4_type=V-type(Left)  p5_type=V-type(Left)  p6_type=V-type(Left)  p7_type=V-type(Left)  p8_type=V-type(Left)  p9_type=V-type(Left)  p10_type=V-type(Left)  p11_type=V-type(Left)  p12_type=V-type(Left)  p13_type=V-type(Left)  p14_type=V-type(Left)  p15_type=V-type(Left)  p16_type=V-type(Left)  I_port_shunt_resistance=1e9
  Status : Subsystem
  Status1 : Subsystem
  Sum : Sum  Inputs=|++
  Sum1 : Sum  Inputs=|++
  Switch{,1..3} (4 alike) : Switch
  Terminator{,1..7} (8 alike) : Terminator
  TestSequenceCommands : Subsystem  AncestorBlock=TestSeq_slave_lib/TestSequenceCommands
  Three-Phase Source1 : powerlib/Electrical Sources/Three-Phase Source  Voltage=115000  PhaseAngle=0  Frequency=60  InternalConnection=Yg  SpecifyImpedance=on  Resistance=0.8929  Inductance=16.58e-3  ShortCircuitLevel=2000e6  BaseVoltage=115000  XRratio=100  BusType=swing  Pref=0  Qref=0  Qmin=-inf  Qmax=inf
  Trigg_machine : Subsystem
  Trigg_machine1 : Subsystem
  XFR DYg-30 HIL1 : transformer_lib/XFR DYg-30 HIL  Rating=50000  Vp=115000  Vs=13800  Z=6  XR=30
  XFR DYg-30 HIL2 : transformer_lib/XFR DYg-30 HIL  Rating=50000  Vp=115000  Vs=13800  Z=6  XR=30
  XFR DYg-30 HIL3 : transformer_lib/XFR DYg-30 HIL  Rating=50000  Vp=115000  Vs=13800  Z=6  XR=30
  isOddOrEven : Subsystem
  isOddOrEven1 : Subsystem
  selected_Irms_a : Subsystem
  A_F3 : PMIOPort  Port=1  Side=Right
  B_F3 : PMIOPort  Port=2  Side=Right
  C_F3 : PMIOPort  Port=3  Side=Right
  A_F2 : PMIOPort  Port=4  Side=Right
  B_F2 : PMIOPort  Port=5  Side=Right
  C_F2 : PMIOPort  Port=6  Side=Right
  A_F1 : PMIOPort  Port=7  Side=Right
  B_F1 : PMIOPort  Port=8  Side=Right
  C_F1 : PMIOPort  Port=9  Side=Right
  HWCtrl_TestSeq : Outport
  wires:
  2X MCB - Genset_signal_scaling - 3.5MVA/1 -> Bus Creator4/1  "NGCHP_ScaledSignals"
  Genset_signal_scaling - 4MVA/1 -> Bus Creator4/2  "Diesel_ScaledSignals"
  [CMBNE_SGNLS] -> Bus Selector4/1, Bus Selector2/1, Bus Selector1/1  "MCB"
  Bus Selector4/3 -> 2X MCB - Genset_signal_scaling - 3.5MVA/3  "<Rotor speed  wm (pu)>"
  Bus Selector4/2 -> 2X MCB - Genset_signal_scaling - 3.5MVA/2  "<F3_PCC>"
  Bus Selector4/1 -> 2X MCB - Genset_signal_scaling - 3.5MVA/1  "<cb_ms>"
  Bus Creator4/1 -> Banshee_HWCtrl_IOs/1(ScaledSignals)
  Bus Selector1/3 -> Genset_signal_scaling - 4MVA/3  "<Rotor speed  wm (pu)>"
  Bus Selector1/2 -> Genset_signal_scaling - 4MVA/2  "<F1_PCC>"
  Bus Selector1/1 -> Genset_signal_scaling - 4MVA/1  "<cb_ms>"
  CMBNE_SGNLS/1 -> OpComm2/1
  OpComm2/1 -> [CMBNE_SGNLS]
  SEL751 - SignalScaling/1 -> Bus Creator4/3  "SEL751_ScaledSignals"
  Bus Selector2/2 -> SEL751 - SignalScaling/2  "<F2_PCC>"
  Bus Selector2/1 -> SEL751 - SignalScaling/1  "<F1_PCC>"
  Bus Selector2/3 -> SEL751 - SignalScaling/3  "<F3_PCC>"
  Bus Selector4/4 -> 2X MCB - Genset_signal_scaling - 3.5MVA/4  "<F3_CB_3>"
  [CMBNE_SGNLS] -> Banshee_HWCtrl_IOs/2(CMBNE_SGNLS)
  Mux3/1 -> OpWriteFile2/1, OpWriteFile1/1
  Trigg_machine/1(Trig_odd) -> OpTrigger/1
  Trigg_machine/2(Trig_even) -> OpTrigger1/1
  Constant1/1 -> OpTrigger/2
  Constant4/1 -> OpTrigger1/2
  isOddOrEven/1(isOdd) -> Trigg_machine/2(Odd), Switch/2
  isOddOrEven/2(isEven) -> Trigg_machine/3(Even), Switch1/2
  Switch/1 -> OpWriteFile1/2
  Switch1/1 -> OpWriteFile2/2
  Constant2/1 -> Sum/2
  Sum/1 -> Switch1/3, Switch/3
  Number of seconds of recording/1(file suffix) -> Switch/1, Switch1/1, Sum/1, isOddOrEven/1(Index)  "File suffix"
  Bus Selector8/1 -> Trigg_machine/1(Write)  "<record_rms_signals>"
  OpWriteFile1/2 -> Terminator/1
  OpWriteFile2/2 -> Terminator1/1
  Bus Selector/1 -> PQFV/1  "<F1_PCC>"
  Bus Selector/2 -> PQFV2/1  "<F3_PCC>"
  Bus Selector7/1 -> Mux/2
  Bus Selector5/1 -> Mux/1
  Bus Selector3/1 -> Mux3/1  "DIESEL_CHP_DATA"
  Mux/1 -> Mux3/2  "F1_F3_DATA"
  CONSOLE/1 -> OpComm1/1
  OpComm1/1 -> [CONSOLE]
  [CONSOLE] -> Bus Selector8/1
  Mux2/1 -> OpWriteFile5/1, OpWriteFile4/1
  Trigg_machine1/1(Trig_odd) -> OpTrigger2/1
  Trigg_machine1/2(Trig_even) -> OpTrigger3/1
  Constant3/1 -> OpTrigger2/2
  Constant6/1 -> OpTrigger3/2
  isOddOrEven1/1(isOdd) -> Trigg_machine1/2(Odd), Switch2/2
  isOddOrEven1/2(isEven) -> Trigg_machine1/3(Even), Switch3/2
  Switch2/1 -> OpWriteFile4/2
  Switch3/1 -> OpWriteFile5/2
  Constant5/1 -> Sum1/2
  Sum1/1 -> Switch3/3, Switch2/3
  Number of seconds of recording1/1(file suffix) -> Switch2/1, Switch3/1, Sum1/1, isOddOrEven1/1(Index)  "File suffix"
  Bus Selector10/1 -> Trigg_machine1/1(Write)  "<record_inst_signals>"
  OpWriteFile4/2 -> Terminator2/1
  OpWriteFile5/2 -> Terminator3/1
  [CONSOLE] -> Bus Selector10/1
  [CMBNE_SGNLS] -> Bus Selector16/1, Bus Selector3/1, selected_Irms_a/1(CMBNE_SGNLS), Bus Selector21/1, Bus Selector/1
  Feeder_CB/1 -> Terminator4/1
  [CONSOLE] -> Bus Selector12/1
  [CONSOLE] -> Bus Selector13/1
  [CONSOLE] -> Bus Selector14/1
  [CONSOLE] -> Bus Selector15/1
  Feeder_CB1/1 -> Terminator5/1
  Feeder_CB2/1 -> Terminator6/1
  Feeder_CB3/1 -> Terminator7/1
  Bus Selector12/1 -> Logical Operator1/2  "<Logic_trip>"
  Bus Selector13/1 -> Feeder_CB3/1  "<Grid_F3>"
  Bus Selector14/1 -> Feeder_CB2/1  "<Grid_F2>"
  Bus Selector15/1 -> Feeder_CB1/1  "<Grid_F1>"
  [CMBNE_SGNLS] -> Bus Selector19/1, Bus Selector6/1, Bus Selector11/1, Bus Selector9/1
  Bus Selector9/1 -> Mux2/1
  [CONSOLE] -> Bus Creator1/1  "SC_Signal"
  Bus Selector11/1 -> Status/1(SEL751)  "<Status>"
  Bus Selector11/2 -> Status/2(CBX03)  "<Status>"
  Bus Selector11/3 -> Status/3(GCB)  "<Status>"
  Bus Selector6/1 -> Status1/1(SEL751)  "<Status>"
  Bus Selector6/2 -> Status1/2(CBX03)  "<Status>"
  Bus Selector6/3 -> Status1/3(GCB)  "<Status>"
  Status/1(o) -> Mux2/2
  Status1/1(o) -> Mux2/3
  PQFV/1 -> Bus Selector17/1, Bus Selector5/1
  PQFV2/1 -> Bus Selector18/1, Bus Selector7/1
  Bus Selector16/1 -> Mux1/1
  Bus Selector17/1 -> Mux1/2
  Bus Selector18/1 -> Mux1/3
  Mux1/1 -> [kW_kVAR]
  [kW_kVAR] -> Mux2/4
  Bus Selector19/1 -> Mux2/5
  Bus Selector21/1 -> Mux3/3
  Memory1/1 -> HWCtrl_TestSeq/1
  Banshee_HWCtrl_IOs/1(WoodwardBias) -> Memory3/1
  TestSequenceCommands/1(TestSeqData) -> Memory2/1
  Memory3/1 -> Bus Creator/2  "HWCtrl"
  Memory2/1 -> Bus Creator/1, Bus Selector20/1  "TestSeq"
  Bus Creator/1 -> Memory1/1
  selected_Irms_a/1(Irms_a) -> Mux3/4
  Bus Creator1/1 -> Banshee_HWCtrl_IOs/3(DTT_like_Signal)
  Bus Selector20/1 -> [cut_grid_pwr]  "<Cut_Grid_Power>"
  [cut_grid_pwr] -> Bus Creator1/2  "cut_grid_pwr"
  [cut_grid_pwr] -> Logical Operator/1
  Logical Operator/1 -> Logical Operator1/1
  Logical Operator1/1 -> Bus Creator2/1  "Logic_trip"
  Bus Creator2/1 -> Feeder_CB/1
  connections:
  500kcmil-Mutual3/LConn3 -- Feeder_CB/RConn3
  500kcmil-Mutual3/LConn1 -- Feeder_CB/RConn1
  500kcmil-Mutual3/LConn2 -- Feeder_CB/RConn2
  SSN Interface Block (3ph)3/LConn2 -- 500kcmil-Mutual1/LConn2 -- 500kcmil-Mutual3/RConn2
  SSN Interface Block (3ph)3/LConn1 -- 500kcmil-Mutual1/LConn1 -- 500kcmil-Mutual3/RConn1
  SSN Interface Block (3ph)3/LConn3 -- 500kcmil-Mutual1/LConn3 -- 500kcmil-Mutual3/RConn3
  500kcmil-Mutual4/RConn3 -- Feeder_CB/LConn3
  500kcmil-Mutual4/RConn2 -- Feeder_CB/LConn2
  500kcmil-Mutual4/RConn1 -- Feeder_CB/LConn1
  500kcmil-Mutual4/LConn3 -- Three-Phase Source1/RConn3
  500kcmil-Mutual4/LConn1 -- Three-Phase Source1/RConn1
  500kcmil-Mutual4/LConn2 -- Three-Phase Source1/RConn2
  500kcmil-Mutual2/RConn2 -- XFR DYg-30 HIL1/LConn2
  500kcmil-Mutual2/RConn1 -- XFR DYg-30 HIL1/LConn1
  500kcmil-Mutual2/RConn3 -- XFR DYg-30 HIL1/LConn3
  500kcmil-Mutual5/RConn2 -- XFR DYg-30 HIL2/LConn2
  500kcmil-Mutual5/RConn1 -- XFR DYg-30 HIL2/LConn1
  500kcmil-Mutual5/RConn3 -- XFR DYg-30 HIL2/LConn3
  500kcmil-Mutual1/RConn3 -- XFR DYg-30 HIL3/LConn3
  500kcmil-Mutual1/RConn2 -- XFR DYg-30 HIL3/LConn2
  500kcmil-Mutual1/RConn1 -- XFR DYg-30 HIL3/LConn1
  SSN Interface Block (3ph)3/RConn1 -- 500kcmil-Mutual5/LConn1 -- 500kcmil-Mutual2/LConn1
  SSN Interface Block (3ph)3/RConn2 -- 500kcmil-Mutual5/LConn2 -- 500kcmil-Mutual2/LConn2
  SSN Interface Block (3ph)3/RConn3 -- 500kcmil-Mutual5/LConn3 -- 500kcmil-Mutual2/LConn3
  XFR DYg-30 HIL2/RConn1 -- Feeder_CB3/LConn1
  XFR DYg-30 HIL2/RConn2 -- Feeder_CB3/LConn2
  XFR DYg-30 HIL2/RConn3 -- Feeder_CB3/LConn3
  XFR DYg-30 HIL1/RConn3 -- Feeder_CB2/LConn3
  XFR DYg-30 HIL1/RConn2 -- Feeder_CB2/LConn2
  XFR DYg-30 HIL1/RConn1 -- Feeder_CB2/LConn1
  Feeder_CB1/LConn3 -- XFR DYg-30 HIL3/RConn3
  Feeder_CB1/LConn2 -- XFR DYg-30 HIL3/RConn2
  Feeder_CB1/LConn1 -- XFR DYg-30 HIL3/RConn1
  500kcmil-Mutual6/LConn2 -- Feeder_CB3/RConn2
  500kcmil-Mutual6/LConn3 -- Feeder_CB3/RConn3
  500kcmil-Mutual6/LConn1 -- Feeder_CB3/RConn1
  500kcmil-Mutual7/LConn2 -- Feeder_CB2/RConn2
  500kcmil-Mutual7/LConn3 -- Feeder_CB2/RConn3
  500kcmil-Mutual7/LConn1 -- Feeder_CB2/RConn1
  500kcmil-Mutual8/LConn1 -- Feeder_CB1/RConn1
  500kcmil-Mutual8/LConn2 -- Feeder_CB1/RConn2
  500kcmil-Mutual8/LConn3 -- Feeder_CB1/RConn3
  B_F1/RConn1 -- 500kcmil-Mutual8/RConn2
  C_F1/RConn1 -- 500kcmil-Mutual8/RConn3
  A_F1/RConn1 -- 500kcmil-Mutual8/RConn1
  B_F2/RConn1 -- 500kcmil-Mutual7/RConn2
  A_F2/RConn1 -- 500kcmil-Mutual7/RConn1
  C_F2/RConn1 -- 500kcmil-Mutual7/RConn3
  B_F3/RConn1 -- 500kcmil-Mutual6/RConn2
  A_F3/RConn1 -- 500kcmil-Mutual6/RConn1
  C_F3/RConn1 -- 500kcmil-Mutual6/RConn3

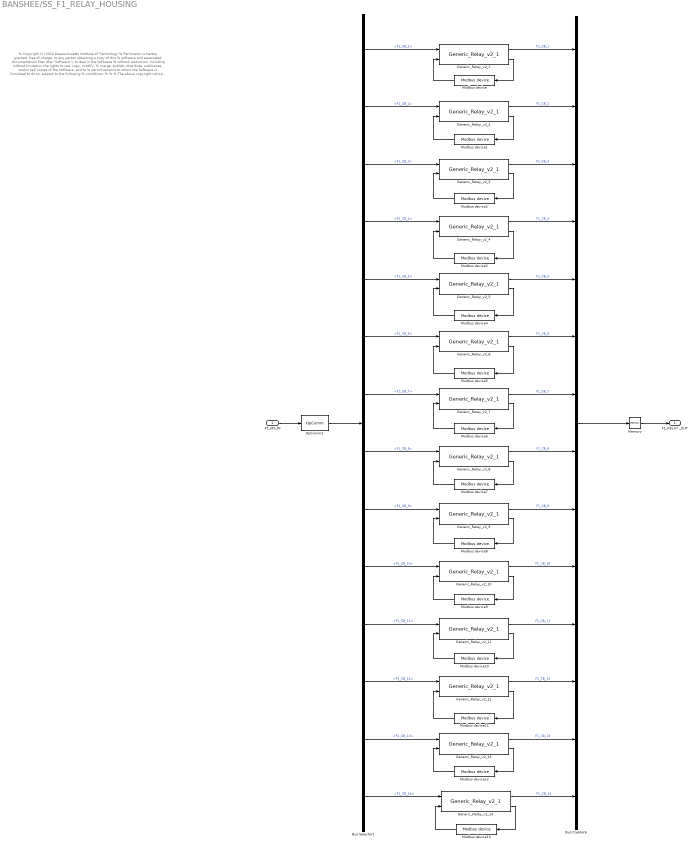
== system BANSHEE/SS_F1_RELAY_HOUSING ==
  note: % Copyright (c) 2016 Massachusetts Institute of Technology
      | % Permission is hereby granted, free of charge, to any person obtaining a copy of this
      | % software and associated documentation files (the "Software"), to deal in the Software
      | % without restriction, including without limitation the rights to use, copy, modify,
      | % merge, publish, distribute, sublicense, and/or sell copies of the Software, and to
      | % permit persons to whom the Software is furnished to do so, subject to the following
      | % conditions:
      | %
      | %
      | % The above copyright notice and this permission notice shall be included in
      | % all copies or substantial portions of the Software.
      | %
      | % THE SOFTWARE IS PROVIDED "AS IS", WITHOUT WARRANTY OF ANY KIND, EXPRESS OR IMPLIED,
      | % INCLUDING BUT NOT LIMITED TO THE WARRANTIES OF MERCHANTABILITY, FITNESS FOR A
      | % PARTICULAR PURPOSE AND NONINFRINGEMENT. IN NO EVENT SHALL THE AUTHORS OR COPYRIGHT
      | % HOLDERS BE LIABLE FOR ANY CLAIM, DAMAGES OR OTHER LIABILITY, WHETHER IN AN ACTION
      | % OF CONTRACT, TORT OR OTHERWISE, ARISING FROM, OUT OF OR IN CONNECTION WITH THE
      | % SOFTWARE OR THE USE OR OTHER DEALINGS IN THE SOFTWARE.
      | %
      | %
      | %%
  F1_MS_IN : Inport
  Bus Creator6 : BusCreator  Inputs=14
  Bus Selector1 : BusSelector  OutputSignals=CB_DATA.F1_CB_1,CB_DATA.F1_CB_2,CB_DATA.F1_CB_3,CB_DATA.F1_CB_4,CB_DATA.F1_CB_5,CB_DATA.F1_CB_6,CB_DATA.F1_CB_7,CB_DATA.F1_CB_8,CB_DATA.F1_CB_9,CB_DATA.F1_CB_10,CB_DATA.F1_CB_11,CB_DATA.F1_CB_12,CB_DATA.F1_CB_13,CB_DATA.F1_CB_14
  Generic_Relay_v2_1 : relay_modbus_lib/Generic_Relay_v2_1  Ts=Ts  relay_settings=[F1(1,:)]
  Generic_Relay_v2_10 : relay_modbus_lib/Generic_Relay_v2_1  Ts=Ts  relay_settings=[F1(10,:)]
  Generic_Relay_v2_11 : relay_modbus_lib/Generic_Relay_v2_1  Ts=Ts  relay_settings=[F1(11,:)]
  Generic_Relay_v2_12 : relay_modbus_lib/Generic_Relay_v2_1  Ts=Ts  relay_settings=[F1(12,:)]
  Generic_Relay_v2_13 : relay_modbus_lib/Generic_Relay_v2_1  Ts=Ts  relay_settings=[F1(13,:)]
  Generic_Relay_v2_14 : relay_modbus_lib/Generic_Relay_v2_1  Ts=Ts  relay_settings=[F1(14,:)]
  Generic_Relay_v2_2 : relay_modbus_lib/Generic_Relay_v2_1  Ts=Ts  relay_settings=[F1(2,:)]
  Generic_Relay_v2_3 : relay_modbus_lib/Generic_Relay_v2_1  Ts=Ts  relay_settings=[F1(3,:)]
  Generic_Relay_v2_4 : relay_modbus_lib/Generic_Relay_v2_1  Ts=Ts  relay_settings=[F1(4,:)]
  Generic_Relay_v2_5 : relay_modbus_lib/Generic_Relay_v2_1  Ts=Ts  relay_settings=[F1(5,:)]
  Generic_Relay_v2_6 : relay_modbus_lib/Generic_Relay_v2_1  Ts=Ts  relay_settings=[F1(6,:)]
  Generic_Relay_v2_7 : relay_modbus_lib/Generic_Relay_v2_1  Ts=Ts  relay_settings=[F1(7,:)]
  Generic_Relay_v2_8 : relay_modbus_lib/Generic_Relay_v2_1  Ts=Ts  relay_settings=[F1(8,:)]
  Generic_Relay_v2_9 : relay_modbus_lib/Generic_Relay_v2_1  Ts=Ts  relay_settings=[F1(9,:)]
  Memory : Memory
  Modbus device : rtio_generic_modbus/Modbus device  conf_name=F1_relay_cfg1.opal  conf_name_mask=F1_relay_cfg1.xls  sample_time=Ts
  Modbus device1 : rtio_generic_modbus/Modbus device  conf_name=F1_relay_cfg2.opal  conf_name_mask=F1_relay_cfg2.xls  sample_time=Ts
  Modbus device10 : rtio_generic_modbus/Modbus device  conf_name=F1_relay_cfg11.opal  conf_name_mask=F1_relay_cfg11.xls  sample_time=Ts
  Modbus device11 : rtio_generic_modbus/Modbus device  conf_name=F1_relay_cfg12.opal  conf_name_mask=F1_relay_cfg12.xls  sample_time=Ts
  Modbus device12 : rtio_generic_modbus/Modbus device  conf_name=F1_relay_cfg13.opal  conf_name_mask=F1_relay_cfg13.xls  sample_time=Ts
  Modbus device13 : rtio_generic_modbus/Modbus device  conf_name=F1_relay_cfg14.opal  conf_name_mask=F1_relay_cfg14.xls  sample_time=Ts
  Modbus device2 : rtio_generic_modbus/Modbus device  conf_name=F1_relay_cfg3.opal  conf_name_mask=F1_relay_cfg3.xls  sample_time=Ts
  Modbus device3 : rtio_generic_modbus/Modbus device  conf_name=F1_relay_cfg4.opal  conf_name_mask=F1_relay_cfg4.xls  sample_time=Ts
  Modbus device4 : rtio_generic_modbus/Modbus device  conf_name=F1_relay_cfg5.opal  conf_name_mask=F1_relay_cfg5.xls  sample_time=Ts
  Modbus device5 : rtio_generic_modbus/Modbus device  conf_name=F1_relay_cfg6.opal  conf_name_mask=F1_relay_cfg6.xls  sample_time=Ts
  Modbus device6 : rtio_generic_modbus/Modbus device  conf_name=F1_relay_cfg7.opal  conf_name_mask=F1_relay_cfg7.xls  sample_time=Ts
  Modbus device7 : rtio_generic_modbus/Modbus device  conf_name=F1_relay_cfg8.opal  conf_name_mask=F1_relay_cfg8.xls  sample_time=Ts
  Modbus device8 : rtio_generic_modbus/Modbus device  conf_name=F1_relay_cfg9.opal  conf_name_mask=F1_relay_cfg9.xls  sample_time=Ts
  Modbus device9 : rtio_generic_modbus/Modbus device  conf_name=F1_relay_cfg10.opal  conf_name_mask=F1_relay_cfg10.xls  sample_time=Ts
  OpComm2 : rtlab/OpComm  nbport=1  groupe_acq=1  subsys_rate=0  st=0  Synchronization=on  Interpolation=on  Threshold=1.0  Missed_Data=off  Sim_Time=off  Samples=off  dynSigOut=off  from_console=0  warning_done=off  writeOpCommFile=off  Offset=off
  F1_RELAY _OUT : Outport
  wires:
  OpComm2/1 -> Bus Selector1/1
  Modbus device12/1 -> Generic_Relay_v2_13/2
  Generic_Relay_v2_13/2 -> Modbus device12/1
  Modbus device11/1 -> Generic_Relay_v2_12/2
  Generic_Relay_v2_12/2 -> Modbus device11/1
  Modbus device10/1 -> Generic_Relay_v2_11/2
  Generic_Relay_v2_11/2 -> Modbus device10/1
  Modbus device9/1 -> Generic_Relay_v2_10/2
  Generic_Relay_v2_10/2 -> Modbus device9/1
  Modbus device8/1 -> Generic_Relay_v2_9/2
  Generic_Relay_v2_9/2 -> Modbus device8/1
  Modbus device7/1 -> Generic_Relay_v2_8/2
  Generic_Relay_v2_8/2 -> Modbus device7/1
  Modbus device6/1 -> Generic_Relay_v2_7/2
  Generic_Relay_v2_7/2 -> Modbus device6/1
  Modbus device5/1 -> Generic_Relay_v2_6/2
  Generic_Relay_v2_6/2 -> Modbus device5/1
  Modbus device4/1 -> Generic_Relay_v2_5/2
  Generic_Relay_v2_5/2 -> Modbus device4/1
  Modbus device3/1 -> Generic_Relay_v2_4/2
  Generic_Relay_v2_4/2 -> Modbus device3/1
  Modbus device2/1 -> Generic_Relay_v2_3/2
  Generic_Relay_v2_3/2 -> Modbus device2/1
  Generic_Relay_v2_2/2 -> Modbus device1/1
  Modbus device1/1 -> Generic_Relay_v2_2/2
  Generic_Relay_v2_1/2 -> Modbus device/1
  Modbus device/1 -> Generic_Relay_v2_1/2
  F1_MS_IN/1 -> OpComm2/1
  Bus Selector1/1 -> Generic_Relay_v2_1/1  "<F1_CB_1>"
  Generic_Relay_v2_1/1 -> Bus Creator6/1  "F1_CB_1"
  Bus Creator6/1 -> Memory/1
  Bus Selector1/2 -> Generic_Relay_v2_2/1  "<F1_CB_2>"
  Generic_Relay_v2_2/1 -> Bus Creator6/2  "F1_CB_2"
  Bus Selector1/3 -> Generic_Relay_v2_3/1  "<F1_CB_3>"
  Bus Selector1/4 -> Generic_Relay_v2_4/1  "<F1_CB_4>"
  Bus Selector1/5 -> Generic_Relay_v2_5/1  "<F1_CB_5>"
  Bus Selector1/6 -> Generic_Relay_v2_6/1  "<F1_CB_6>"
  Bus Selector1/7 -> Generic_Relay_v2_7/1  "<F1_CB_7>"
  Bus Selector1/8 -> Generic_Relay_v2_8/1  "<F1_CB_8>"
  Bus Selector1/9 -> Generic_Relay_v2_9/1  "<F1_CB_9>"
  Bus Selector1/10 -> Generic_Relay_v2_10/1  "<F1_CB_10>"
  Bus Selector1/11 -> Generic_Relay_v2_11/1  "<F1_CB_11>"
  Bus Selector1/12 -> Generic_Relay_v2_12/1  "<F1_CB_12>"
  Bus Selector1/13 -> Generic_Relay_v2_13/1  "<F1_CB_13>"
  Generic_Relay_v2_13/1 -> Bus Creator6/13  "F1_CB_13"
  Generic_Relay_v2_12/1 -> Bus Creator6/12  "F1_CB_12"
  Generic_Relay_v2_11/1 -> Bus Creator6/11  "F1_CB_11"
  Generic_Relay_v2_10/1 -> Bus Creator6/10  "F1_CB_10"
  Generic_Relay_v2_9/1 -> Bus Creator6/9  "F1_CB_9"
  Generic_Relay_v2_8/1 -> Bus Creator6/8  "F1_CB_8"
  Generic_Relay_v2_7/1 -> Bus Creator6/7  "F1_CB_7"
  Generic_Relay_v2_6/1 -> Bus Creator6/6  "F1_CB_6"
  Generic_Relay_v2_5/1 -> Bus Creator6/5  "F1_CB_5"
  Generic_Relay_v2_4/1 -> Bus Creator6/4  "F1_CB_4"
  Generic_Relay_v2_3/1 -> Bus Creator6/3  "F1_CB_3"
  Modbus device13/1 -> Generic_Relay_v2_14/2
  Generic_Relay_v2_14/2 -> Modbus device13/1
  Generic_Relay_v2_14/1 -> Bus Creator6/14  "F1_CB_14"
  Bus Selector1/14 -> Generic_Relay_v2_14/1  "<F1_CB_14>"
  Memory/1 -> F1_RELAY _OUT/1
